simulink model "ldpc_encoder_model"  (R2020b)
settings: Solver=FixedStepDiscrete  StartTime=0.0  StopTime=1  RelTol=1e-3
values from neighbouring files (symbols this model uses):
  codeword = [message; fliplr(parity_bits')']    [bch_encoder.m]    (also in bch_lfsr_encode_test.m; interleave.m = zeros(size(message)); interleave_test.m = interleave(message); ldpc_encode.m = [message parity]')
libraries: hdlsllib x2, simulink x1, commsink2 x1
settings Model: DataTypeOverride=Off  Creator=wardo  LastModifiedBy=wardo
settings SolverCC: AutoInsertRateTranBlk=on
settings DataIOCC: LimitDataPoints=on  SaveOutput=off  SaveTime=off
settings OptimizationCC: BlockReduction=off  ConditionallyExecuteInputs=off  DefaultParameterBehavior=Inlined  LifeSpan=inf
settings DebuggingCC: AlgebraicLoopMsg=error  SingleTaskRateTransMsg=error  AllowSymbolicDim=off  StrictBusMsg=ErrorOnBusTreatedAsVector  SFUnexpectedBacktrackingDiag=warning  SFNoUnconditionalDefaultTransitionDiag=warning  SFExecutionAtInitializationDiag=none  ArithmeticOperatorsInVariantConditions=warning
settings HardwareCC: ProdBitPerPointer=32  ProdBitPerSizeT=32  ProdBitPerPtrDiffT=32  ProdLargestAtomicFloat=None  ProdIntDivRoundTo=Undefined  ProdEndianess=Unspecified  ProdWordSize=32  ProdHWDeviceType=ASIC/FPGA->ASIC/FPGA  ProdEqTarget=off
settings SFSimCC: SimUseLocalCustomCode=off  CustomCodeUndefinedFunction=UseInterfaceOnly
settings RTWCC: RTWUseLocalCustomCode=off
settings CodeAppCC: StateflowObjectComments=on
settings GRTTargetCC: TargetLangStandard=C89/C90 (ANSI)
settings ConfigComp: CovScope=ReferencedModels  CovMetricSettings=dw  CovSaveCumulativeToWorkspaceVar=on  CovSaveSingleToWorkspaceVar=on  CovExternalEMLEnable=off  CovSFcnEnable=off

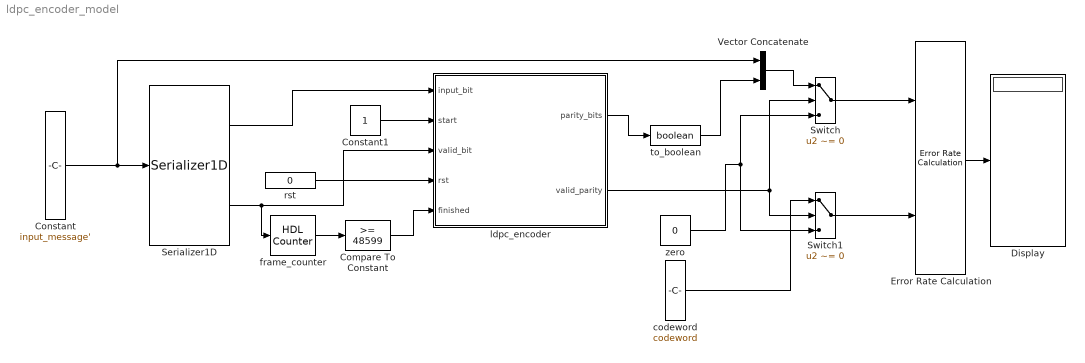
== system ldpc_encoder_model ==
  Compare To Constant : simulink/Logic and Bit Operations/Compare To Constant  relop=>=  const=48599  OutDataTypeStr=boolean
  Constant : Constant  Value=input_message'  VectorParams1D=off  OutDataTypeStr=boolean  SampleTime=1
  Constant1 : Constant
  Display : Display
  Error Rate Calculation : commsink2/Error Rate Calculation  N=0  st_delay=0  cp_mode=Entire frame  subframe=[]  PMode=Port  WsName=ErrorVec  RsMode2=off  stop=off  numErr=100  maxBits=1e6
      settings: SourceProductName=Communications Toolbox
  Serializer1D : hdlsllib/HDL Operations/Serializer1D  Ratio=48600  IdleCycles=0  validIn=off  startOut=off  validOut=on  inputDataDimensions=-1  inputSampleTime=-1  inputSignalType=auto
      settings: SourceProductBaseCode=SL
  Switch : Switch  Criteria=u2 ~= 0
  Switch1 : Switch  Criteria=u2 ~= 0
  Vector Concatenate : Concatenate
  codeword : Constant  Value=codeword  OutDataTypeStr=boolean  SampleTime=1
  frame_counter : hdlsllib/Sources/HDL Counter  CountType=Count limited  CountInit=0  CountStep=1  CountMax=48600  CountFromType=Initial value  CountFrom=0  CountResetPort=off  CountLoadPort=off  CountEnbPort=on  CountDirPort=off  CountDataType=Unsigned  CountWordLen=16  CountFracLen=0  CountSampTime=1
  ldpc_encoder : Subsystem
  rst : Constant  Value=0  OutDataTypeStr=boolean  SampleTime=inf'
  to_boolean : DataTypeConversion  OutDataTypeStr=boolean
  zero : Constant  Value=0  OutDataTypeStr=boolean  SampleTime=1
  wires:
  ldpc_encoder/1(parity_bits) -> to_boolean/1
  Serializer1D/1 -> ldpc_encoder/1(input_bit)
  rst/1 -> ldpc_encoder/4(rst)
  Error Rate Calculation/1 -> Display/1
  frame_counter/1 -> Compare To Constant/1
  Compare To Constant/1 -> ldpc_encoder/5(finished)
  Serializer1D/2 -> frame_counter/1, ldpc_encoder/3(valid_bit)
  Constant/1 -> Vector Concatenate/1, Serializer1D/1
  codeword/1 -> Switch1/1
  Vector Concatenate/1 -> Switch/1
  ldpc_encoder/2(valid_parity) -> Switch1/2, Switch/2
  Switch/1 -> Error Rate Calculation/1
  Switch1/1 -> Error Rate Calculation/2
  zero/1 -> Switch/3, Switch1/3
  to_boolean/1 -> Vector Concatenate/2
  Constant1/1 -> ldpc_encoder/2(start)

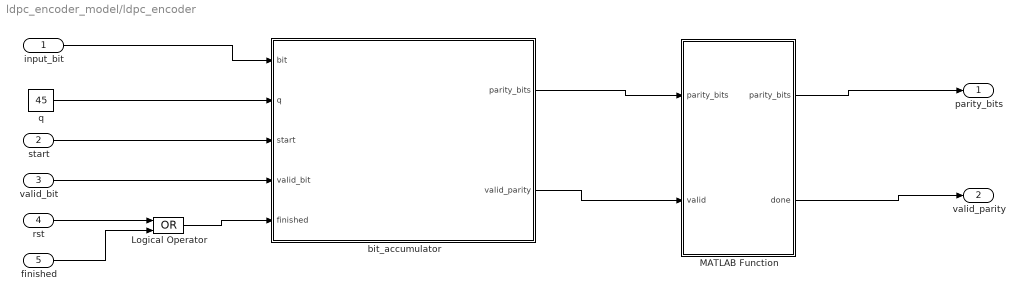
== system ldpc_encoder_model/ldpc_encoder ==
  input_bit : Inport
  start : Inport  Port=2
  valid_bit : Inport  Port=3
  rst : Inport  Port=4
  finished : Inport  Port=5
  Logical Operator : Logic  Operator=OR  AllPortsSameDT=off  OutDataTypeStr=boolean
  MATLAB Function : MATLAB Function  TreatAsAtomicUnit=on
  bit_accumulator : MATLAB Function  TreatAsAtomicUnit=on
  q : Constant  Value=45  OutDataTypeStr=uint32  SampleTime=-1
  parity_bits : Outport  VectorParamsAs1DForOutWhenUnconnected=off
  valid_parity : Outport  Port=2  VectorParamsAs1DForOutWhenUnconnected=off
  wires:
  input_bit/1 -> bit_accumulator/1(bit)
  bit_accumulator/2(valid_parity) -> MATLAB Function/2(valid)
  start/1 -> bit_accumulator/3(start)
  finished/1 -> Logical Operator/2
  rst/1 -> Logical Operator/1
  q/1 -> bit_accumulator/2(q)
  valid_bit/1 -> bit_accumulator/4(valid_bit)
  bit_accumulator/1(parity_bits) -> MATLAB Function/1("parity_bits ")
  MATLAB Function/2(done) -> valid_parity/1
  MATLAB Function/1(parity_bits) -> parity_bits/1
  Logical Operator/1 -> bit_accumulator/5(finished)

== matlab function ldpc_encoder_model/ldpc_encoder/bit_accumulator ==
  settings: fimath=fimath('RoundingMethod', 'Floor','OverflowAction', 'Wrap','ProductMode', 'FullPrecision', 'SumMode', 'FullPrecision')
  data: parity_bits output; bit input; q input; valid_parity output; start input; valid_bit input; finished input
function [parity_bits, valid_parity] = fsm_ldpc_accum_bit(bit, q, start, valid_bit, finished)
%#codegen
primary_parity_bit_addr = [[0 6385 7901 14611 13389 11200 3252 5243 2504 2722 821 7374];
               [1 11359 2698 357 13824 12772 7244 6752 15310 852 2001 11417];
               [2 7862 7977 6321 13612 12197 14449 15137 13860 1708 6399 13444];
               [3 1560 11804 6975 13292 3646 3812 8772 7306 5795 14327 7866];
               [4 7626 11407 14599 9689 1628 2113 10809 9283 1230 15241 4870];
               [5 1610 5699 15876 9446 12515 1400 6303 5411 14181 13925 7358];
               [6 4059 8836 3405 7853 7992 15336 5970 10368 10278 9675 4651];
               [7 4441 3963 9153 2109 12683 7459 12030 12221 629 15212 406];
               [8 6007 8411 5771 3497 543 14202 875 9186 6235 13908 3563];
               [9 3232 6625 4795 546 9781 2071 7312 3399 7250 4932 12652];
               [10 8820 10088 11090 7069 6585 13134 10158 7183 488 7455 9238];
               [11 1903 10818 119 215 7558 11046 10615 11545 14784 7961 15619];
               [12 3655 8736 4917 15874 5129 2134 15944 14768 7150 2692 1469];
               [13 8316 3820 505 8923 6757 806 7957 4216 15589 13244 2622];
               [14 14463 4852 15733 3041 11193 12860 13673 8152 6551 15108 8758]];
second_parity_bit_addr = [[15 3149 11981];
                           [16 13416 6906];
                           [17 13098 13352];
                           [18 2009 14460];
                           [19 7207 4314];
                           [20 3312 3945];
                           [21 4418 6248];
                           [22 2669 13975];
                           [23 7571 9023];
                           [24 14172 2967];
                           [25 7271 7138];
                           [26 6135 13670];
                           [27 7490 14559];
                           [28 8657 2466];
                           [29 8599 12834];
                           [30 3470 3152];
                           [31 13917 4365];
                           [32 6024 13730];
                           [33 10973 14182];
                           [34 2464 13167];
                           [35 5281 15049];
                           [36 1103 1849];
                           [37 2058 1069];
                           [38 9654 6095];
                           [39 14311 7667];
                           [40 15617 8146];
                           [41 4588 11218];
                           [42 13660 6243];
                           [43 8578 7874];
                           [44 11741 2686];
                           [0 1022 1264];
                           [1 12604 9965];
                           [2 8217 2707];
                           [3 3156 11793];
                           [4 354 1514];
                           [5 6978 14058];
                           [6 7922 16079];
                           [7 15087 12138];
                           [8 5053 6470];
                           [9 12687 14932];
                           [10 15458 1763];
                           [11 8121 1721];
                           [12 12431 549];
                           [13 4129 7091];
                           [14 1426 8415];
                           [15 9783 7604];
                           [16 6295 11329];
                           [17 1409 12061];
                           [18 8065 9087];
                           [19 2918 8438];
                           [20 1293 14115];
                           [21 3922 13851];
                           [22 3851 4000];
                           [23 5865 1768];
                           [24 2655 14957];
                           [25 5565 6332];
                           [26 4303 12631];
                           [27 11653 12236];
                           [28 16025 7632];
                           [29 4655 14128];
                           [30 9584 13123];
                           [31 13987 9597];
                           [32 15409 12110];
                           [33 8754 15490];
                           [34 7416 15325];
                           [35 2909 15549];
                           [36 2995 8257];
                           [37 9406 4791];
                           [38 11111 4854];
                           [39 2812 8521];
                           [40 8476 14717];
                           [41 7820 15360];
                           [42 1179 7939];
                           [43 2357 8678];
                           [44 7703 6216];
                           [0 3477 7067];
                           [1 3931 13845];
                           [2 7675 12899];
                           [3 1754 8187];
                           [4 7785 1400];
                           [5 9213 5891];
                           [6 2494 7703];
                           [7 2576 7902];
                           [8 4821 15682];
                           [9 10426 11935];
                           [10 1810 904];
                           [11 11332 9264];
                           [12 11312 3570];
                           [13 14916 2650];
                           [14 7679 7842];
                           [15 6089 13084];
                           [16 3938 2751];
                           [17 8509 4648];
                           [18 12204 8917];
                           [19 5749 12443];
                           [20 12613 4431];
                           [21 1344 4014];
                           [22 8488 13850];
                           [23 1730 14896];
                           [24 14942 7126];
                           [25 14983 8863];
                           [26 6578 8564];
                           [27 4947 396];
                           [28 297 12805];
                           [29 13878 6692];
                           [30 11857 11186];
                           [31 14395 11493];
                           [32 16145 12251];
                           [33 13462 7428];
                           [34 14526 13119];
                           [35 2535 11243];
                           [36 6465 12690];
                           [37 6872 9334];
                           [38 15371 14023];
                           [39 8101 10187];
                           [40 11963 4848];
                           [41 15125 6119];
                           [42 8051 14465];
                           [43 11139 5167];
                           [44 2883 14521]];
num_parity_bits = 16200;
state_iddle    = 0;
state_accum = 1;
one = 1;

persistent moore_state_reg;
if isempty(moore_state_reg)
    moore_state_reg = fi(0, 0, 2, 0);   
end  

persistent parity;
if isempty(parity)
    parity = fi(zeros(num_parity_bits, 1), 0, 1, 0);
end

% Counter used to count from 0 to 359 for each slot of 360 bits
% Counter stores the input bit position in the message modulo 360.
persistent counter;
if isempty(counter)
    counter = fi(0, 0, 9, 0);
end

persistent address_index;
if isempty(address_index)
    address_index = fi(1, 0, 8, 0);
end

switch (moore_state_reg)
    
    case state_iddle 
        parity_bits   = parity;
        valid_parity = false;
        if (~start)
            moore_state_reg(1) = state_iddle;
        else
            moore_state_reg(1) = state_accum;
            % Accumulate first bit
            parity   = fi(zeros(num_parity_bits, 1), 0, 1, 0);
            buffer = primary_parity_bit_addr(1, :) + counter*q;
            adrr = buffer - num_parity_bits .* uint32(buffer >= num_parity_bits);
            parity(adrr+1) = xor(parity(adrr+1), bit);
            counter = fi(counter + 1, 0, 9, 0);
        end

    case state_accum 
        if finished
            valid_parity       = true;
            address_index      = fi(1, 0, 8, 0);
            counter            = fi(0, 0, 9, 0);
            moore_state_reg(1) = state_iddle;
        else
            % Accumulate bit at computed addresses
            if valid_bit
                if address_index <= 15
                    buffer = primary_parity_bit_addr(address_index, :) + counter*q;
                else
                    buffer = second_parity_bit_addr(address_index-15, :) + counter*q;
                end
                adrr = buffer - num_parity_bits .* uint32(buffer >= num_parity_bits);
                parity(adrr+1) = xor(parity(adrr+1), bit);
                if counter == 359
                    address_index = fi(address_index + one, 0, 8, 0);
                end
                counter = fi((counter + one) * (counter + one < 360), 0, 9, 0);
            end
            valid_parity   = false;
        end
        parity_bits        = parity;

    otherwise
        valid_parity = false;
        parity_bits  = parity;      
end

== matlab function ldpc_encoder_model/ldpc_encoder/MATLAB Function ==
  data: parity_bits input; parity_bits output; valid input; done output
function [parity_bits, done] = xor_accum_bits(parity_bits, valid)
%#codegen
done = false;
num_parity_bits = 16200;
if valid    
    for i = 2:num_parity_bits
        parity_bits(i) = xor(parity_bits(i), parity_bits(i-1));
    end
    done = true;
end
